simulink model "moveMotor"  (Simulink 8.2)
settings: Solver=FixedStepDiscrete  StartTime=0.0  StopTime=inf  RelTol=1e-3
libraries: simulink x1
settings Model: Creator=deastman  LastModifiedBy=pvinnako
settings DataIOCC: SignalLoggingSaveFormat=Dataset  SaveOutput=off  DSMLogging=off  SaveTime=off
settings DebuggingCC: StrictBusMsg=Warning

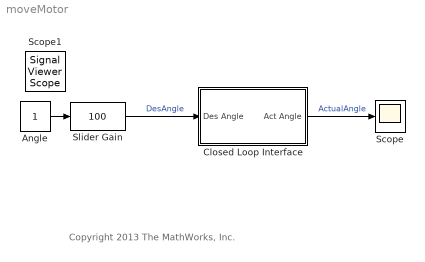
== system moveMotor ==
  note: Copyright 2013 The MathWorks, Inc.
  Angle : Constant
  Closed Loop Interface : Subsystem
  Scope : Scope
  Slider Gain : simulink/Math Operations/Slider Gain  low=-100  gain=100  high=100
  Scope1 : SignalViewerScope  IOType=viewer  RefreshTime=0.035000
      settings: TimeRange=30  YMin=-100  YMax=100
  wires:
  Slider Gain/1 -> Closed Loop Interface/1(Des Angle)  "DesAngle"
  Closed Loop Interface/1(Act Angle) -> Scope/1  "ActualAngle"
  Angle/1 -> Slider Gain/1

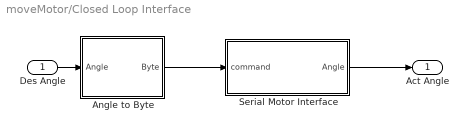
== system moveMotor/Closed Loop Interface ==
  Des Angle : Inport
  Angle to Byte : Subsystem
  Serial Motor Interface : Subsystem  StartFcn=|  StopFcn=|
      StartFcn=|
      | openInstr = instrfind;                           
      | if ~isempty(openInstr)                           
      |   fclose(openInstr);                             
      |   delete(openInstr);                             
      | end                                              
      | clear openInstr                                  
      | s = serial('COM4', 'BaudRate', 9600,'Timeout',5);
      | fopen(s);
      StopFcn=|
      | fclose(s);
      | delete(s);
      | clear s
  Act Angle : Outport
  wires:
  Serial Motor Interface/1(Angle) -> Act Angle/1
  Des Angle/1 -> Angle to Byte/1(Angle)
  Angle to Byte/1(Byte) -> Serial Motor Interface/1(command)

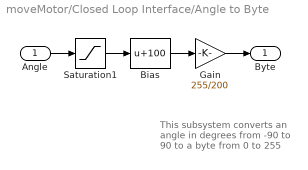
== system moveMotor/Closed Loop Interface/Angle to Byte ==
  note: This subsystem converts an angle
      |  in degrees from -90 to 90 to a byte from 0 to 255
  Angle : Inport
  Bias : Bias  Bias=100
  Gain : Gain  Gain=255/200  OutDataTypeStr=uint8
  Saturation1 : Saturate  UpperLimit=100  LowerLimit=-100
  Byte : Outport
  wires:
  Bias/1 -> Gain/1
  Saturation1/1 -> Bias/1
  Gain/1 -> Byte/1
  Angle/1 -> Saturation1/1

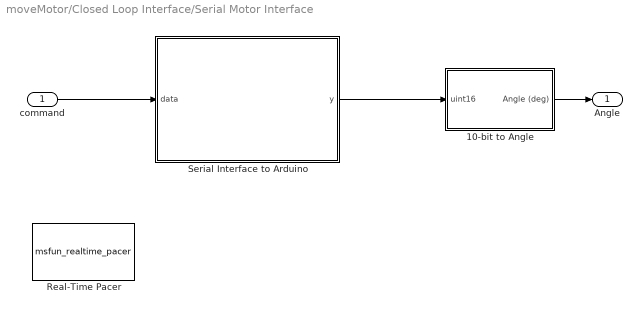
== system moveMotor/Closed Loop Interface/Serial Motor Interface ==
  command : Inport  OutDataTypeStr=uint8  SampleTime=0.01
  10-bit to Angle : Subsystem
  Real-Time Pacer : M-S-Function  FunctionName=msfun_realtime_pacer  Parameters=simTimePerRealTime  mask(RealTime_Pacer){simTimePerRealTime=1}
      mask prompts: simTimePerRealTime "Speedup (Simulation Time / Real Time):"
      mask help:
      | Slow down a simulation to track real (i.e., wall clock) elapsed time.
      |
      | "Speedup" specifies the ratio between simulation time and real time
      | • Speedup = N => N sec. of simulation time per sec. of real time
      | • Speedup can be fractional (e.g., 0.5, 1.3).
      | • Speedup = inf => allow simulation to run at full speed
      |
      | Click on the Help button for details.
      mask Help: web('realtime_pacer_help.html', '-helpbrowser')
      mask Display: fprintf('Real-Time Pacer\nSpeedup = %g', simTimePerRealTime)
  Serial Interface to Arduino : MATLAB Function  TreatAsAtomicUnit=on  SystemSampleTime=1/100
  Angle : Outport
  wires:
  Serial Interface to Arduino/1(y) -> 10-bit to Angle/1(uint16)
  command/1 -> Serial Interface to Arduino/1(data)
  10-bit to Angle/1(Angle (deg)) -> Angle/1

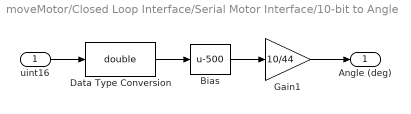
== system moveMotor/Closed Loop Interface/Serial Motor Interface/10-bit to Angle ==
  uint16 : Inport
  Bias : Bias  Bias=-500
  Data Type Conversion : DataTypeConversion  OutDataTypeStr=double
  Gain1 : Gain  Gain=10/44
  Angle (deg) : Outport
  wires:
  Gain1/1 -> Angle (deg)/1
  uint16/1 -> Data Type Conversion/1
  Data Type Conversion/1 -> Bias/1
  Bias/1 -> Gain1/1

== matlab function Closed Loop Interface/Serial Motor Interface/Serial Interface to Arduino ==
  data: data input uint8 size=1; y output int16 size=1
function y = serialFcn(data)

    coder.extrinsic('fread','fwrite','instrfind')
    
    persistent s last
   
    % Declaring parameters
    HEADER = 'A';
    PACKET_SIZE = 4;
    packet = zeros(PACKET_SIZE,1,'int16');
   
    % Initializing the serial object
    if isempty(s)
        s = instrfind;        
        last = int16(0);
    end
    
    % Write data to the serial port  
    fwrite(s,data,'uint8');
    
    % Read data from the serial port
    packet = int16(fread(s, PACKET_SIZE, 'uint8'));
    
    % Check for header and convert two bytes to single int16
    if (packet(1) ~= HEADER)
          y = last;
    else 
          y  = 2^8*packet(3)+packet(2);
          last = y;
    end
% y= 0;
